simulink model "fft_16pt_CRD_simulink_v1"  (R2022b)
settings: Solver=FixedStepAuto  StartTime=0.0  StopTime=inf  RelTol=1e-3
undefined symbols (not defined in the file): j
libraries: dsphdlsigops2 x1
settings Model: Creator=caleb  LastModifiedBy=caleb

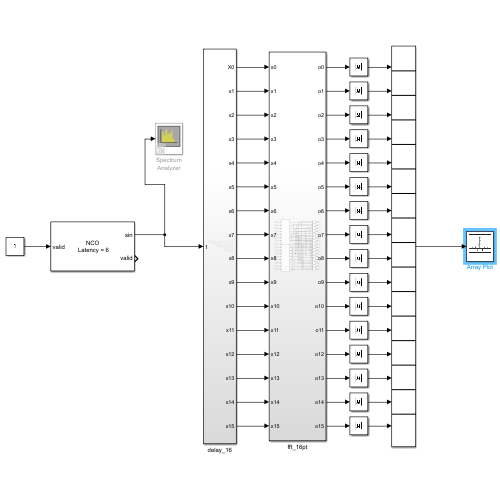
[thumbnail: Simulink's stored preview of the top-level diagram]
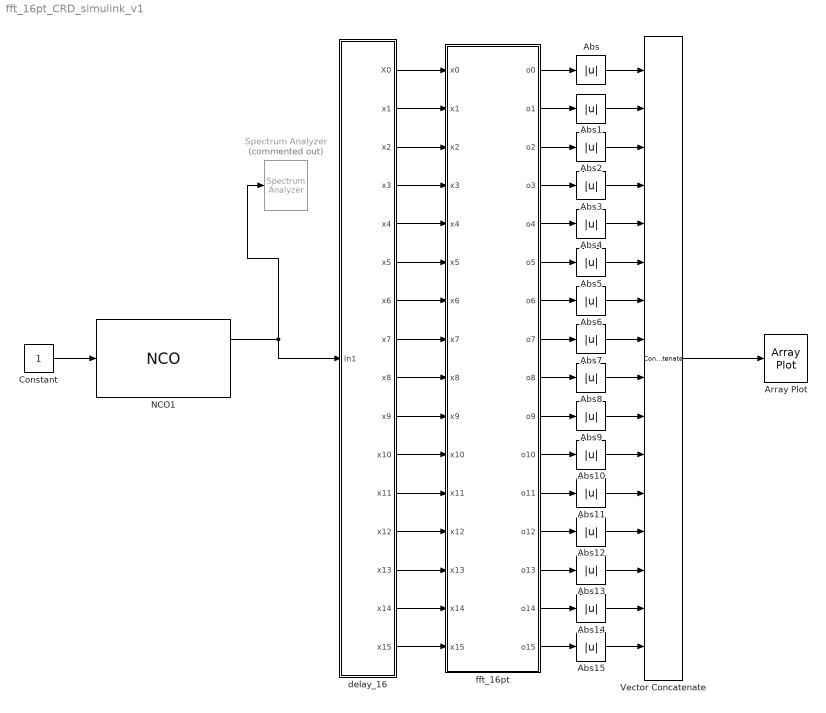
== system fft_16pt_CRD_simulink_v1 ==
  Abs{,1..15} (16 alike) : Abs  SaturateOnIntegerOverflow=off
  Array Plot : ArrayPlot  WindowPosition=[436.000000,111.000000,800.000000,500.000000,]  ScopeFrameLocation=window  YLimits=[-0.961,9.0519]
  Constant : Constant  VectorParams1D=off  OutDataTypeStr=boolean  SampleTime=1/16
  NCO1 : dsphdlsigops2/NCO  PhaseIncrementSource=Property  PhaseIncrement=phIncr  PhaseOffsetSource=Property  PhaseOffset=phOff  DitherSource=Property  NumDitherBits=ditherBits  SamplesPerFrame=1  LUTCompress=off  ResetAction=off  Waveform=Sine  PhasePort=off  SimulateUsing=Code generation  AccumulatorWL=N  PhaseQuantization=off  NumQuantizerAccumulatorBits=Q  OutputDataType=double  OutputWL=16  OutputFL=14
  Spectrum Analyzer : SpectrumAnalyzer  Commented=on
  Vector Concatenate : Concatenate  NumInputs=16
  delay_16 : Subsystem
  fft_16pt : Subsystem
  wires:
  NCO1/1 -> Spectrum Analyzer/1, delay_16/1(In1)
  Constant/1 -> NCO1/1
  delay_16/1(X0) -> fft_16pt/1(x0)
  delay_16/2(x1) -> fft_16pt/2(x1)
  delay_16/3(x2) -> fft_16pt/3(x2)
  delay_16/4(x3) -> fft_16pt/4(x3)
  delay_16/5(x4) -> fft_16pt/5(x4)
  delay_16/6(x5) -> fft_16pt/6(x5)
  delay_16/7(x6) -> fft_16pt/7(x6)
  delay_16/8(x7) -> fft_16pt/8(x7)
  delay_16/9(x8) -> fft_16pt/9(x8)
  delay_16/10(x9) -> fft_16pt/10(x9)
  delay_16/11(x10) -> fft_16pt/11(x10)
  delay_16/12(x11) -> fft_16pt/12(x11)
  delay_16/13(x12) -> fft_16pt/13(x12)
  delay_16/14(x13) -> fft_16pt/14(x13)
  delay_16/15(x14) -> fft_16pt/15(x14)
  delay_16/16(x15) -> fft_16pt/16(x15)
  fft_16pt/1(o0) -> Abs/1
  fft_16pt/2(o1) -> Abs1/1
  fft_16pt/3(o2) -> Abs2/1
  fft_16pt/4(o3) -> Abs3/1
  fft_16pt/5(o4) -> Abs4/1
  fft_16pt/6(o5) -> Abs5/1
  fft_16pt/7(o6) -> Abs6/1
  fft_16pt/8(o7) -> Abs7/1
  fft_16pt/9(o8) -> Abs8/1
  fft_16pt/10(o9) -> Abs9/1
  fft_16pt/11(o10) -> Abs10/1
  fft_16pt/12(o11) -> Abs11/1
  fft_16pt/13(o12) -> Abs12/1
  fft_16pt/14(o13) -> Abs13/1
  fft_16pt/15(o14) -> Abs14/1
  fft_16pt/16(o15) -> Abs15/1
  Abs15/1 -> Vector Concatenate/16
  Abs14/1 -> Vector Concatenate/15
  Abs13/1 -> Vector Concatenate/14
  Abs12/1 -> Vector Concatenate/13
  Abs10/1 -> Vector Concatenate/11
  Abs9/1 -> Vector Concatenate/10
  Abs11/1 -> Vector Concatenate/12
  Abs8/1 -> Vector Concatenate/9
  Abs7/1 -> Vector Concatenate/8
  Abs6/1 -> Vector Concatenate/7
  Abs5/1 -> Vector Concatenate/6
  Abs4/1 -> Vector Concatenate/5
  Abs3/1 -> Vector Concatenate/4
  Abs1/1 -> Vector Concatenate/2
  Abs/1 -> Vector Concatenate/1
  Abs2/1 -> Vector Concatenate/3
  Vector Concatenate/1 -> Array Plot/1

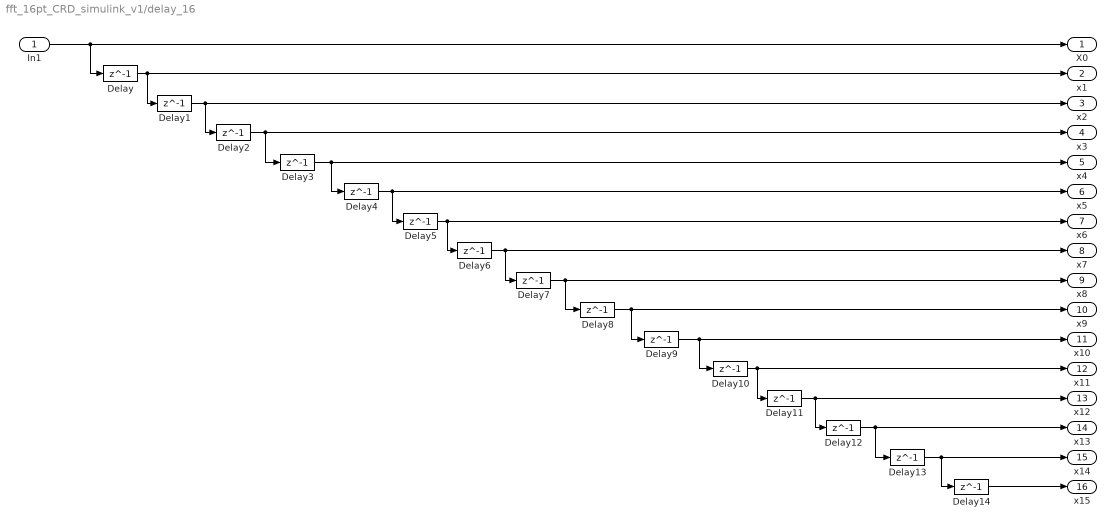
== system fft_16pt_CRD_simulink_v1/delay_16 ==
  In1 : Inport
  Delay{,1..14} (15 alike) : Delay  DelayLength=1  InitialCondition=0  UseCircularBuffer=on
  X0 : Outport
  x1 : Outport  Port=2
  x2 : Outport  Port=3
  x3 : Outport  Port=4
  x4 : Outport  Port=5
  x5 : Outport  Port=6
  x6 : Outport  Port=7
  x7 : Outport  Port=8
  x8 : Outport  Port=9
  x9 : Outport  Port=10
  x10 : Outport  Port=11
  x11 : Outport  Port=12
  x12 : Outport  Port=13
  x13 : Outport  Port=14
  x14 : Outport  Port=15
  x15 : Outport  Port=16
  wires:
  In1/1 -> Delay/1, X0/1
  Delay/1 -> Delay1/1, x1/1
  Delay1/1 -> Delay2/1, x2/1
  Delay2/1 -> Delay3/1, x3/1
  Delay3/1 -> Delay4/1, x4/1
  Delay4/1 -> Delay5/1, x5/1
  Delay7/1 -> x8/1, Delay8/1
  Delay8/1 -> x9/1, Delay9/1
  Delay5/1 -> x6/1, Delay6/1
  Delay6/1 -> x7/1, Delay7/1
  Delay9/1 -> Delay10/1, x10/1
  Delay12/1 -> x13/1, Delay13/1
  Delay13/1 -> x14/1, Delay14/1
  Delay10/1 -> x11/1, Delay11/1
  Delay14/1 -> x15/1
  Delay11/1 -> x12/1, Delay12/1

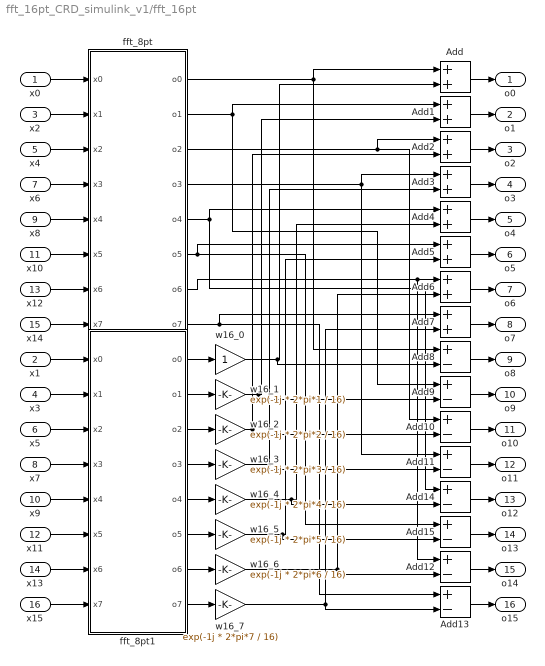
== system fft_16pt_CRD_simulink_v1/fft_16pt ==
  x0 : Inport
  x1 : Inport  Port=2
  x2 : Inport  Port=3
  x3 : Inport  Port=4
  x4 : Inport  Port=5
  x5 : Inport  Port=6
  x6 : Inport  Port=7
  x7 : Inport  Port=8
  x8 : Inport  Port=9
  x9 : Inport  Port=10
  x10 : Inport  Port=11
  x11 : Inport  Port=12
  x12 : Inport  Port=13
  x13 : Inport  Port=14
  x14 : Inport  Port=15
  x15 : Inport  Port=16
  Add{,1..7} (8 alike) : Sum
  Add{8..15} (8 alike) : Sum  Inputs=+-
  fft_8pt : Subsystem
  fft_8pt1 : Subsystem
  w16_0 : Gain
  w16_1 : Gain  Gain=exp(-1j * 2*pi*1 / 16)
  w16_2 : Gain  Gain=exp(-1j * 2*pi*2 / 16)
  w16_3 : Gain  Gain=exp(-1j * 2*pi*3 / 16)
  w16_4 : Gain  Gain=exp(-1j * 2*pi*4 / 16)
  w16_5 : Gain  Gain=exp(-1j * 2*pi*5 / 16)
  w16_6 : Gain  Gain=exp(-1j * 2*pi*6 / 16)
  w16_7 : Gain  Gain=exp(-1j * 2*pi*7 / 16)
  o0 : Outport
  o1 : Outport  Port=2
  o2 : Outport  Port=3
  o3 : Outport  Port=4
  o4 : Outport  Port=5
  o5 : Outport  Port=6
  o6 : Outport  Port=7
  o7 : Outport  Port=8
  o8 : Outport  Port=9
  o9 : Outport  Port=10
  o10 : Outport  Port=11
  o11 : Outport  Port=12
  o12 : Outport  Port=13
  o13 : Outport  Port=14
  o14 : Outport  Port=15
  o15 : Outport  Port=16
  wires:
  fft_8pt1/1(o0) -> w16_0/1
  fft_8pt1/2(o1) -> w16_1/1
  fft_8pt1/3(o2) -> w16_2/1
  fft_8pt1/4(o3) -> w16_3/1
  fft_8pt1/5(o4) -> w16_4/1
  fft_8pt1/6(o5) -> w16_5/1
  fft_8pt1/7(o6) -> w16_6/1
  fft_8pt1/8(o7) -> w16_7/1
  x0/1 -> fft_8pt/1(x0)
  x2/1 -> fft_8pt/2(x1)
  x4/1 -> fft_8pt/3(x2)
  x6/1 -> fft_8pt/4(x3)
  x8/1 -> fft_8pt/5(x4)
  x10/1 -> fft_8pt/6(x5)
  x12/1 -> fft_8pt/7(x6)
  x14/1 -> fft_8pt/8(x7)
  x1/1 -> fft_8pt1/1(x0)
  x3/1 -> fft_8pt1/2(x1)
  x5/1 -> fft_8pt1/3(x2)
  x7/1 -> fft_8pt1/4(x3)
  x9/1 -> fft_8pt1/5(x4)
  x11/1 -> fft_8pt1/6(x5)
  x13/1 -> fft_8pt1/7(x6)
  x15/1 -> fft_8pt1/8(x7)
  Add/1 -> o0/1
  Add1/1 -> o1/1
  Add3/1 -> o3/1
  Add7/1 -> o7/1
  Add9/1 -> o9/1
  Add11/1 -> o11/1
  Add10/1 -> o10/1
  Add14/1 -> o12/1
  Add15/1 -> o13/1
  Add12/1 -> o14/1
  Add13/1 -> o15/1
  Add8/1 -> o8/1
  Add6/1 -> o6/1
  Add5/1 -> o5/1
  Add4/1 -> o4/1
  Add2/1 -> o2/1
  fft_8pt/1(o0) -> Add8/1, Add/1
  w16_0/1 -> Add8/2, Add/2
  fft_8pt/2(o1) -> Add1/1, Add9/1
  w16_1/1 -> Add9/2, Add1/2
  fft_8pt/3(o2) -> Add10/1, Add2/1
  w16_2/1 -> Add2/2, Add10/2
  fft_8pt/4(o3) -> Add3/1, Add11/1
  w16_3/1 -> Add3/2, Add11/2
  fft_8pt/5(o4) -> Add4/1, Add14/1
  w16_4/1 -> Add14/2, Add4/2
  fft_8pt/6(o5) -> Add15/1, Add5/1
  w16_5/1 -> Add15/2, Add5/2
  fft_8pt/7(o6) -> Add6/1, Add12/1
  w16_6/1 -> Add6/2, Add12/2
  fft_8pt/8(o7) -> Add13/1, Add7/1
  w16_7/1 -> Add7/2, Add13/2

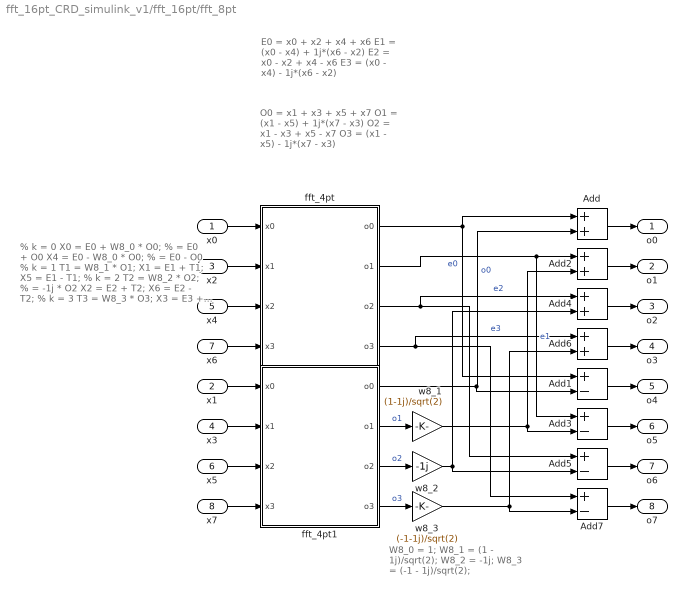
== system fft_16pt_CRD_simulink_v1/fft_16pt/fft_8pt ==
  note: E0 = x0 + x2 + x4 + x6
      | E1 = (x0 - x4) + 1j*(x6 - x2)
      | E2 = x0 - x2 + x4 - x6
      | E3 = (x0 - x4) - 1j*(x6 - x2)
  note: O0 = x1 + x3 + x5 + x7
      | O1 = (x1 - x5) + 1j*(x7 - x3)
      | O2 = x1 - x3 + x5 - x7
      | O3 = (x1 - x5) - 1j*(x7 - x3)
  note: W8_0 = 1;
      | W8_1 = (1 - 1j)/sqrt(2);
      | W8_2 = -1j;
      | W8_3 = (-1 - 1j)/sqrt(2);
  note: % k = 0
      | X0 = E0 + W8_0 * O0;   % = E0 + O0
      | X4 = E0 - W8_0 * O0;   % = E0 - O0
      |
      | % k = 1
      | T1 = W8_1 * O1;
      | X1 = E1 + T1;
      | X5 = E1 - T1;
      |
      | % k = 2
      | T2 = W8_2 * O2;        % = -1j * O2
      | X2 = E2 + T2;
      | X6 = E2 - T2;
      |
      | % k = 3
      | T3 = W8_3 * O3;
      | X3 = E3 + T3;
      | X7 = E3 - T3;
  x0 : Inport
  x1 : Inport  Port=2
  x2 : Inport  Port=3
  x3 : Inport  Port=4
  x4 : Inport  Port=5
  x5 : Inport  Port=6
  x6 : Inport  Port=7
  x7 : Inport  Port=8
  Add{,2,4,6} (4 alike) : Sum
  Add{1,3,5,7} (4 alike) : Sum  Inputs=+-
  fft_4pt : Subsystem
  fft_4pt1 : Subsystem
  w8_1 : Gain  Gain=(1-1j)/sqrt(2)
  w8_2 : Gain  Gain=-1j
  w8_3 : Gain  Gain=(-1-1j)/sqrt(2)
  o0 : Outport
  o1 : Outport  Port=2
  o2 : Outport  Port=3
  o3 : Outport  Port=4
  o4 : Outport  Port=5
  o5 : Outport  Port=6
  o6 : Outport  Port=7
  o7 : Outport  Port=8
  wires:
  x0/1 -> fft_4pt/1(x0)
  x2/1 -> fft_4pt/2(x1)
  x4/1 -> fft_4pt/3(x2)
  x6/1 -> fft_4pt/4(x3)
  x1/1 -> fft_4pt1/1(x0)
  x3/1 -> fft_4pt1/2(x1)
  x5/1 -> fft_4pt1/3(x2)
  x7/1 -> fft_4pt1/4(x3)
  fft_4pt/1(o0) -> Add1/1, Add/1  "e0"
  fft_4pt/2(o1) -> Add3/1, Add2/1  "e1"
  fft_4pt/3(o2) -> Add5/1, Add4/1  "e2"
  fft_4pt/4(o3) -> Add7/1, Add6/1  "e3"
  fft_4pt1/1(o0) -> Add1/2, Add/2  "o0"
  fft_4pt1/2(o1) -> w8_1/1  "o1"
  fft_4pt1/3(o2) -> w8_2/1  "o2"
  fft_4pt1/4(o3) -> w8_3/1  "o3"
  Add/1 -> o0/1
  Add1/1 -> o4/1
  w8_1/1 -> Add3/2, Add2/2
  w8_2/1 -> Add4/2, Add5/2
  w8_3/1 -> Add7/2, Add6/2
  Add2/1 -> o1/1
  Add4/1 -> o2/1
  Add6/1 -> o3/1
  Add3/1 -> o5/1
  Add5/1 -> o6/1
  Add7/1 -> o7/1

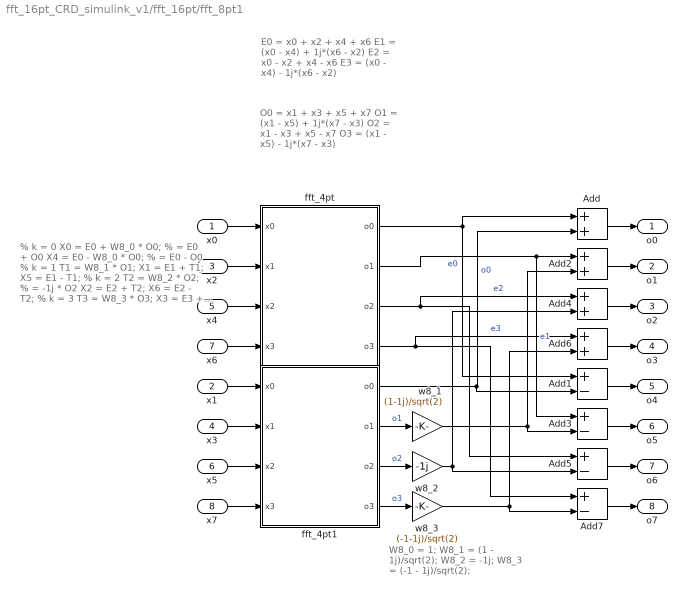
== system fft_16pt_CRD_simulink_v1/fft_16pt/fft_8pt1 ==
  note: E0 = x0 + x2 + x4 + x6
      | E1 = (x0 - x4) + 1j*(x6 - x2)
      | E2 = x0 - x2 + x4 - x6
      | E3 = (x0 - x4) - 1j*(x6 - x2)
  note: O0 = x1 + x3 + x5 + x7
      | O1 = (x1 - x5) + 1j*(x7 - x3)
      | O2 = x1 - x3 + x5 - x7
      | O3 = (x1 - x5) - 1j*(x7 - x3)
  note: W8_0 = 1;
      | W8_1 = (1 - 1j)/sqrt(2);
      | W8_2 = -1j;
      | W8_3 = (-1 - 1j)/sqrt(2);
  note: % k = 0
      | X0 = E0 + W8_0 * O0;   % = E0 + O0
      | X4 = E0 - W8_0 * O0;   % = E0 - O0
      |
      | % k = 1
      | T1 = W8_1 * O1;
      | X1 = E1 + T1;
      | X5 = E1 - T1;
      |
      | % k = 2
      | T2 = W8_2 * O2;        % = -1j * O2
      | X2 = E2 + T2;
      | X6 = E2 - T2;
      |
      | % k = 3
      | T3 = W8_3 * O3;
      | X3 = E3 + T3;
      | X7 = E3 - T3;
  x0 : Inport
  x1 : Inport  Port=2
  x2 : Inport  Port=3
  x3 : Inport  Port=4
  x4 : Inport  Port=5
  x5 : Inport  Port=6
  x6 : Inport  Port=7
  x7 : Inport  Port=8
  Add{,2,4,6} (4 alike) : Sum
  Add{1,3,5,7} (4 alike) : Sum  Inputs=+-
  fft_4pt : Subsystem
  fft_4pt1 : Subsystem
  w8_1 : Gain  Gain=(1-1j)/sqrt(2)
  w8_2 : Gain  Gain=-1j
  w8_3 : Gain  Gain=(-1-1j)/sqrt(2)
  o0 : Outport
  o1 : Outport  Port=2
  o2 : Outport  Port=3
  o3 : Outport  Port=4
  o4 : Outport  Port=5
  o5 : Outport  Port=6
  o6 : Outport  Port=7
  o7 : Outport  Port=8
  wires:
  x0/1 -> fft_4pt/1(x0)
  x2/1 -> fft_4pt/2(x1)
  x4/1 -> fft_4pt/3(x2)
  x6/1 -> fft_4pt/4(x3)
  x1/1 -> fft_4pt1/1(x0)
  x3/1 -> fft_4pt1/2(x1)
  x5/1 -> fft_4pt1/3(x2)
  x7/1 -> fft_4pt1/4(x3)
  fft_4pt/1(o0) -> Add1/1, Add/1  "e0"
  fft_4pt/2(o1) -> Add3/1, Add2/1  "e1"
  fft_4pt/3(o2) -> Add5/1, Add4/1  "e2"
  fft_4pt/4(o3) -> Add7/1, Add6/1  "e3"
  fft_4pt1/1(o0) -> Add1/2, Add/2  "o0"
  fft_4pt1/2(o1) -> w8_1/1  "o1"
  fft_4pt1/3(o2) -> w8_2/1  "o2"
  fft_4pt1/4(o3) -> w8_3/1  "o3"
  Add/1 -> o0/1
  Add1/1 -> o4/1
  w8_1/1 -> Add3/2, Add2/2
  w8_2/1 -> Add4/2, Add5/2
  w8_3/1 -> Add7/2, Add6/2
  Add2/1 -> o1/1
  Add4/1 -> o2/1
  Add6/1 -> o3/1
  Add3/1 -> o5/1
  Add5/1 -> o6/1
  Add7/1 -> o7/1

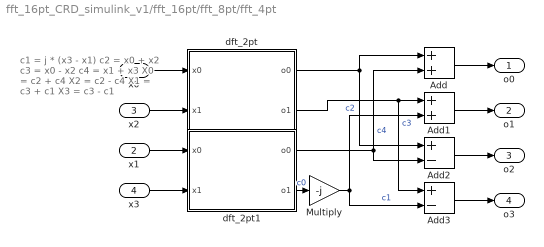
== system fft_16pt_CRD_simulink_v1/fft_16pt/fft_8pt/fft_4pt ==
  note: c1 =  j * (x3 - x1)
      | c2 =  x0 + x2
      | c3 =  x0 - x2
      | c4 =  x1 + x3
      |
      | X0 = c2 + c4
      | X2 = c2 - c4
      | X1 = c3 + c1
      | X3 = c3 - c1
  x0 : Inport
  x1 : Inport  Port=2
  x2 : Inport  Port=3
  x3 : Inport  Port=4
  Add : Sum
  Add1 : Sum
  Add2 : Sum  Inputs=+-
  Add3 : Sum  Inputs=+-
  Multiply : Gain  Gain=-j
  dft_2pt : Subsystem
  dft_2pt1 : Subsystem
  o0 : Outport
  o1 : Outport  Port=2
  o2 : Outport  Port=3
  o3 : Outport  Port=4
  wires:
  x0/1 -> dft_2pt/1(x0)
  x2/1 -> dft_2pt/2(x1)
  x1/1 -> dft_2pt1/1(x0)
  x3/1 -> dft_2pt1/2(x1)
  dft_2pt1/2(o1) -> Multiply/1  "c0"
  dft_2pt/1(o0) -> Add/1, Add2/1  "c2"
  dft_2pt/2(o1) -> Add3/1, Add1/1  "c3"
  dft_2pt1/1(o0) -> Add2/2, Add/2  "c4"
  Multiply/1 -> Add1/2, Add3/2  "c1"
  Add/1 -> o0/1
  Add1/1 -> o1/1
  Add2/1 -> o2/1
  Add3/1 -> o3/1

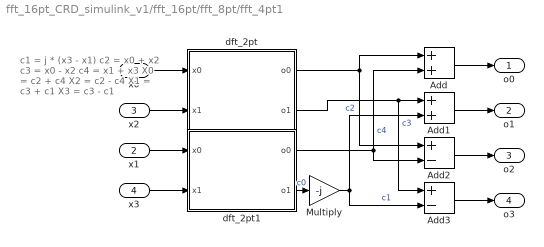
== system fft_16pt_CRD_simulink_v1/fft_16pt/fft_8pt/fft_4pt1 ==
  note: c1 =  j * (x3 - x1)
      | c2 =  x0 + x2
      | c3 =  x0 - x2
      | c4 =  x1 + x3
      |
      | X0 = c2 + c4
      | X2 = c2 - c4
      | X1 = c3 + c1
      | X3 = c3 - c1
  x0 : Inport
  x1 : Inport  Port=2
  x2 : Inport  Port=3
  x3 : Inport  Port=4
  Add : Sum
  Add1 : Sum
  Add2 : Sum  Inputs=+-
  Add3 : Sum  Inputs=+-
  Multiply : Gain  Gain=-j
  dft_2pt : Subsystem
  dft_2pt1 : Subsystem
  o0 : Outport
  o1 : Outport  Port=2
  o2 : Outport  Port=3
  o3 : Outport  Port=4
  wires:
  x0/1 -> dft_2pt/1(x0)
  x2/1 -> dft_2pt/2(x1)
  x1/1 -> dft_2pt1/1(x0)
  x3/1 -> dft_2pt1/2(x1)
  dft_2pt1/2(o1) -> Multiply/1  "c0"
  dft_2pt/1(o0) -> Add/1, Add2/1  "c2"
  dft_2pt/2(o1) -> Add3/1, Add1/1  "c3"
  dft_2pt1/1(o0) -> Add2/2, Add/2  "c4"
  Multiply/1 -> Add1/2, Add3/2  "c1"
  Add/1 -> o0/1
  Add1/1 -> o1/1
  Add2/1 -> o2/1
  Add3/1 -> o3/1

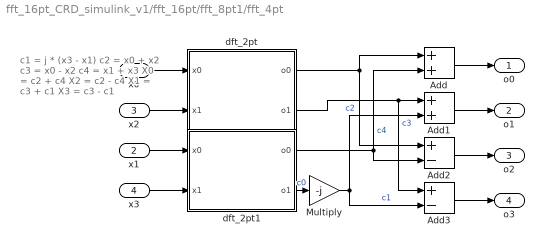
== system fft_16pt_CRD_simulink_v1/fft_16pt/fft_8pt1/fft_4pt ==
  note: c1 =  j * (x3 - x1)
      | c2 =  x0 + x2
      | c3 =  x0 - x2
      | c4 =  x1 + x3
      |
      | X0 = c2 + c4
      | X2 = c2 - c4
      | X1 = c3 + c1
      | X3 = c3 - c1
  x0 : Inport
  x1 : Inport  Port=2
  x2 : Inport  Port=3
  x3 : Inport  Port=4
  Add : Sum
  Add1 : Sum
  Add2 : Sum  Inputs=+-
  Add3 : Sum  Inputs=+-
  Multiply : Gain  Gain=-j
  dft_2pt : Subsystem
  dft_2pt1 : Subsystem
  o0 : Outport
  o1 : Outport  Port=2
  o2 : Outport  Port=3
  o3 : Outport  Port=4
  wires:
  x0/1 -> dft_2pt/1(x0)
  x2/1 -> dft_2pt/2(x1)
  x1/1 -> dft_2pt1/1(x0)
  x3/1 -> dft_2pt1/2(x1)
  dft_2pt1/2(o1) -> Multiply/1  "c0"
  dft_2pt/1(o0) -> Add/1, Add2/1  "c2"
  dft_2pt/2(o1) -> Add3/1, Add1/1  "c3"
  dft_2pt1/1(o0) -> Add2/2, Add/2  "c4"
  Multiply/1 -> Add1/2, Add3/2  "c1"
  Add/1 -> o0/1
  Add1/1 -> o1/1
  Add2/1 -> o2/1
  Add3/1 -> o3/1

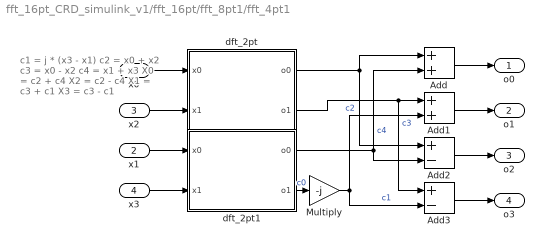
== system fft_16pt_CRD_simulink_v1/fft_16pt/fft_8pt1/fft_4pt1 ==
  note: c1 =  j * (x3 - x1)
      | c2 =  x0 + x2
      | c3 =  x0 - x2
      | c4 =  x1 + x3
      |
      | X0 = c2 + c4
      | X2 = c2 - c4
      | X1 = c3 + c1
      | X3 = c3 - c1
  x0 : Inport
  x1 : Inport  Port=2
  x2 : Inport  Port=3
  x3 : Inport  Port=4
  Add : Sum
  Add1 : Sum
  Add2 : Sum  Inputs=+-
  Add3 : Sum  Inputs=+-
  Multiply : Gain  Gain=-j
  dft_2pt : Subsystem
  dft_2pt1 : Subsystem
  o0 : Outport
  o1 : Outport  Port=2
  o2 : Outport  Port=3
  o3 : Outport  Port=4
  wires:
  x0/1 -> dft_2pt/1(x0)
  x2/1 -> dft_2pt/2(x1)
  x1/1 -> dft_2pt1/1(x0)
  x3/1 -> dft_2pt1/2(x1)
  dft_2pt1/2(o1) -> Multiply/1  "c0"
  dft_2pt/1(o0) -> Add/1, Add2/1  "c2"
  dft_2pt/2(o1) -> Add3/1, Add1/1  "c3"
  dft_2pt1/1(o0) -> Add2/2, Add/2  "c4"
  Multiply/1 -> Add1/2, Add3/2  "c1"
  Add/1 -> o0/1
  Add1/1 -> o1/1
  Add2/1 -> o2/1
  Add3/1 -> o3/1

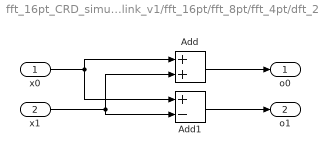
== system fft_16pt_CRD_simulink_v1/fft_16pt/fft_8pt/fft_4pt/dft_2pt ==
  x0 : Inport
  x1 : Inport  Port=2
  Add : Sum
  Add1 : Sum  Inputs=+-
  o0 : Outport
  o1 : Outport  Port=2
  wires:
  x0/1 -> Add1/1, Add/1
  x1/1 -> Add/2, Add1/2
  Add/1 -> o0/1
  Add1/1 -> o1/1

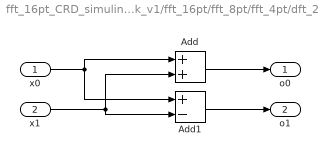
== system fft_16pt_CRD_simulink_v1/fft_16pt/fft_8pt/fft_4pt/dft_2pt1 ==
  x0 : Inport
  x1 : Inport  Port=2
  Add : Sum
  Add1 : Sum  Inputs=+-
  o0 : Outport
  o1 : Outport  Port=2
  wires:
  x0/1 -> Add1/1, Add/1
  x1/1 -> Add/2, Add1/2
  Add/1 -> o0/1
  Add1/1 -> o1/1

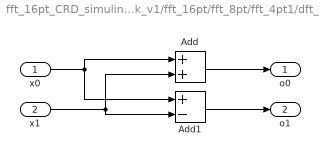
== system fft_16pt_CRD_simulink_v1/fft_16pt/fft_8pt/fft_4pt1/dft_2pt ==
  x0 : Inport
  x1 : Inport  Port=2
  Add : Sum
  Add1 : Sum  Inputs=+-
  o0 : Outport
  o1 : Outport  Port=2
  wires:
  x0/1 -> Add1/1, Add/1
  x1/1 -> Add/2, Add1/2
  Add/1 -> o0/1
  Add1/1 -> o1/1

== system fft_16pt_CRD_simulink_v1/fft_16pt/fft_8pt/fft_4pt1/dft_2pt1 ==
  x0 : Inport
  x1 : Inport  Port=2
  Add : Sum
  Add1 : Sum  Inputs=+-
  o0 : Outport
  o1 : Outport  Port=2
  wires:
  x0/1 -> Add1/1, Add/1
  x1/1 -> Add/2, Add1/2
  Add/1 -> o0/1
  Add1/1 -> o1/1

== system fft_16pt_CRD_simulink_v1/fft_16pt/fft_8pt1/fft_4pt/dft_2pt ==
  x0 : Inport
  x1 : Inport  Port=2
  Add : Sum
  Add1 : Sum  Inputs=+-
  o0 : Outport
  o1 : Outport  Port=2
  wires:
  x0/1 -> Add1/1, Add/1
  x1/1 -> Add/2, Add1/2
  Add/1 -> o0/1
  Add1/1 -> o1/1

== system fft_16pt_CRD_simulink_v1/fft_16pt/fft_8pt1/fft_4pt/dft_2pt1 ==
  x0 : Inport
  x1 : Inport  Port=2
  Add : Sum
  Add1 : Sum  Inputs=+-
  o0 : Outport
  o1 : Outport  Port=2
  wires:
  x0/1 -> Add1/1, Add/1
  x1/1 -> Add/2, Add1/2
  Add/1 -> o0/1
  Add1/1 -> o1/1

== system fft_16pt_CRD_simulink_v1/fft_16pt/fft_8pt1/fft_4pt1/dft_2pt ==
  x0 : Inport
  x1 : Inport  Port=2
  Add : Sum
  Add1 : Sum  Inputs=+-
  o0 : Outport
  o1 : Outport  Port=2
  wires:
  x0/1 -> Add1/1, Add/1
  x1/1 -> Add/2, Add1/2
  Add/1 -> o0/1
  Add1/1 -> o1/1

== system fft_16pt_CRD_simulink_v1/fft_16pt/fft_8pt1/fft_4pt1/dft_2pt1 ==
  x0 : Inport
  x1 : Inport  Port=2
  Add : Sum
  Add1 : Sum  Inputs=+-
  o0 : Outport
  o1 : Outport  Port=2
  wires:
  x0/1 -> Add1/1, Add/1
  x1/1 -> Add/2, Add1/2
  Add/1 -> o0/1
  Add1/1 -> o1/1
